simulink model "SDS_brk_cbc_v1"  (R2018b)
settings: Solver=ode1  StartTime=0.0  StopTime=Inf  FixedStep=0.001  RelTol=1e-3
PostLoadFcn:
  | , if any(exist('dsrtsu_mdlpostloadfcn', 'file') == [2, 3, 6]), try dsrtsu_mdlpostloadfcn('Execute', bdroot); catch fprintf('Error in PostLoadFcn (dsrtsu_mdlpostloadfcn) for model "%s":\n %s\n', bdroot, lasterr); end, end,
libraries: rtican x11, simulink x5
(part 3 of 4)

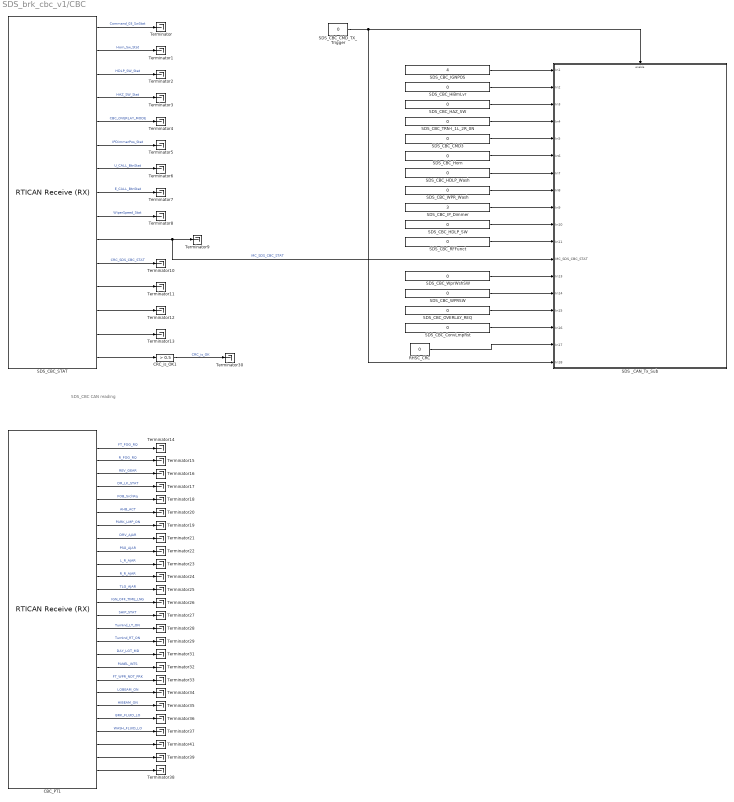
== system SDS_brk_cbc_v1/CBC ==
  note: SDS_CBC CAN reading
  CBC_PT1 : rtican/RTICAN Receive (RX)   Reserved1=[]  Reserved2=[]  Reserved3=[]  Reserved4=[]  SfcnMessage=[]  Msg_Struct=[]  BoardTypeNo=[]  BoardNo=[]  ChannelNo=[]  Parameters=[]  DialogFcn=[]  UnitName=[]  Revision=[]  UnitValues=[]  DSProperties=struct('RTI',struct('Version',uint32(5),'BlockType',struct('isSLSource',uint8(1),'isSLSink',uint8(1),'isHWSource',uint8(0),'isHWSink',uint8(0),'isSetup',uint8(0),'isInline',uint8(1),'isNonInline',uint8(0),'isInterrupt',uint8(0),'isChannelwise',uint8(0)),'IOBoardType','RTICAN','UnitType','MESSAGE','Identifier','RX','DialogType','MSVC','BlockSet','RTICAN','SlaveProcessor','CAN'))  RTIBlockInterface=struct('OutputPortsWidth',int32([1 1 1 1 1 1 1 1 1 1 1 1 1 1 1 1 1 1 1 1 1 1 1 1 1 1]),'OutputPortsActive',ones(1,26),'OutputPortsName',{{'FT_FOG_RQ','R_FOG_RQ','REV_GEAR','DR_LK_STAT','FOB_SrchRq','AHB_ACT','PARK_LMP_ON','DRV_AJAR','PSG_AJAR','L_R_AJAR','R_R_AJAR','TLG_AJAR','IGN_OFF_TIME_LNG','SHIP_STAT','TurnInd_LT_ON','TurnInd_RT_ON','DAY_LGT_MD','PANEL_INTS','FT_WPR_NOT_PRK','LOBEAM_ON','HIBEAM_ON','BRK_FLUID_LO','WASH_FLUID_LO',['RX status'],['RX time'],['RX delta time']}},'OutputPortsDataType',{{'SS_DOUBLE','SS_DOUBLE','SS_DOUBLE','SS_DOUBLE','SS_DOUBLE','SS_DOUBLE','SS_DOUBLE','SS_DOUBLE','SS_DOUBLE','SS_DOUBLE','SS_DOUBLE','SS_DOUBLE','SS_DOUBLE','SS_DOUBLE','SS_DOUBLE','SS_DOUBLE','SS_DOUBLE','SS_DOUBLE','SS_DOUBLE','SS_DOUBLE','SS_DOUBLE','SS_DOUBLE','SS_DOUBLE','SS_DOUBLE','SS_DOUBLE','SS_DOUBLE'}},'OutputPortsLabel',{{'FT_FOG_RQ','R_FOG_RQ','REV_GEAR','DR_LK_STAT','FOB_SrchRq','AHB_ACT','PARK_LMP_ON','DRV_AJAR','PSG_AJAR','L_R_AJAR','R_R_AJAR','TLG_AJAR','IGN_OFF_TIME_LNG','SHIP_STAT','TurnInd_LT_ON','TurnInd_RT_ON','DAY_LGT_MD','PANEL_INTS','FT_WPR_NOT_PRK','LOBEAM_ON','HIBEAM_ON','BRK_FLUID_LO','WASH_FLUID_LO','','',''}},'OutputPortsLabelMode','ON','InputPortsWidth',int32(0),'InputPortsActive',0,'DialogFcn','rtican_message_interface_gui','BlockDisplay',{{'','center'}},'IconTransparency','on','ParameterTunableNames',{{}},'InitLevel',3,'BlockName',struct('Token',{{'CBC_PT1'}}),'SampleTime',{{0}},'TriggerPort',{{'none'}},'EnablePort',{{'none'}})  RTIBlockParameters=struct('BoardTypeNo',{{1,'OFF',[]}},'BoardNo',{{1,'ON',[1 16]}},'ChannelNo',{{1,'ON',[1 2]}},'Parameters',{{struct('DataFileSupport',struct('DataFileSelectedMaster',1,'DataFileSelectedLocal',1,'DataFileName',['c:\intrepidcs\pacifica dbc\e4a_r4_ccan_cr11690_mod.dbc|'],'DataFileDate',{{{['26-Feb-2019 09:25:05']}}},'SelectedFile',['..\..\..\..\..\intrepidcs\pacifica dbc\e4a_r4_ccan_cr11690_mod.dbc']),'Options',struct('StatusSelected',1,'TimeSelected',1,'DeltaTimeSelected',1,'BytePortSelected',0,'MessageLengthSelected',0,'TriggerPort',struct('Selected',0,'TriggerType',0),'UserCoding',struct('Selected',0,'InterfaceFile','UserDecodingFile','FcnName','Message_CRC_Decoder','InportSelected',0,'InportWidth',1,'OutportSelected',1,'OutportWidth',1),'EnablePortSelected',0,'SignalOnPortnameSelected',1,'UseRXService',0),'Message',struct('MsgOnBlocknameSelected',1,'MsgName','CBC_PT1','MsgIdFormat',0,'MsgId',820,'MsgLength',8,'NumSignals',23,'SampleTime',0,'Signal',struct('SgnName',{'FT_FOG_RQ','R_FOG_RQ','REV_GEAR','DR_LK_STAT','FOB_SrchRq','AHB_ACT','PARK_LMP_ON','DRV_AJAR','PSG_AJAR','L_R_AJAR','R_R_AJAR','TLG_AJAR','IGN_OFF_TIME_LNG','SHIP_STAT','TurnInd_LT_ON','TurnInd_RT_ON','DAY_LGT_MD','PANEL_INTS','FT_WPR_NOT_PRK','LOBEAM_ON','HIBEAM_ON','BRK_FLUID_LO','WASH_FLUID_LO'},'SgnStartBit',{2,3,4,5,8,14,16,17,18,19,20,22,24,28,30,31,40,48,56,57,58,62,63},'SgnLength',{1,1,1,2,2,1,1,1,1,1,1,1,12,2,1,1,1,8,1,1,1,1,1},'SgnType',{0,0,0,0,0,0,0,0,0,0,0,0,0,0,0,0,0,0,0,0,0,0,0},'ModeValue',{-1,-1,-1,-1,-1,-1,-1,-1,-1,-1,-1,-1,-1,-1,-1,-1,-1,-1,-1,-1,-1,-1,-1},'DataType',{0,0,0,0,0,0,0,0,0,0,0,0,0,0,0,0,0,0,0,0,0,0,0},'ByteLayout',{0,0,0,0,0,0,0,0,0,0,0,0,2,0,0,0,0,0,0,0,0,0,0},'Factor',{1,1,1,1,1,1,1,1,1,1,1,1,1,1,1,1,1,2^-1,1,1,1,1,1},'Offset',{0,0,0,0,0,0,0,0,0,0,0,0,0,0,0,0,0,0,0,0,0,0,0},'SgnComment',{{['Front fog request; off=[0], on=[1]']},{['Rear fog request; [0] = off, [1] = on']},{['Reverse Gear (manual trans)']},{['Door lock status']},{['FOB search request']},{['Automatic high beam active']},{['Parklamps are on; off=[0], on=[1]']},{['Driver door ajar (1 = Door Ajar)']},{['Passenger door ajar']},{['Left rear door ajar']},{['Right rear door ajar']},{['Trunk/Liftgate ajar']},{['Time since last ignition on (long)']},{['Shipping status']},{['Turn indication left is on']},{['Turn indication right is on']},{['Day light brightness mode; Night=[0], Day=[1]']},{['Panel-/display intensity']},{['Front wiper outside park position']},{['Low beam is on; off=[0], on=[1]']},{['High beam is on; off=[0], on=[1]']},{['Low brake fluid warning; low = [1]']},{['Low washer fluid warning (1=Fluid is low)']}},'SgnUnit',{'','','','','','','','','','','','','min','','','','','%','','','','',''},'Min',{0,0,0,0,0,0,0,0,0,0,0,0,0,0,0,0,0,0,0,0,0,0,0},'Max',{0,0,0,0,0,0,0,0,0,0,0,0,4080,0,0,0,0,100,0,0,0,0,0},'SLDataType',{'SS_DOUBLE','SS_DOUBLE','SS_DOUBLE','SS_DOUBLE','SS_DOUBLE','SS_DOUBLE','SS_DOUBLE','SS_DOUBLE','SS_DOUBLE','SS_DOUBLE','SS_DOUBLE','SS_DOUBLE','SS_DOUBLE','SS_DOUBLE','SS_DOUBLE','SS_DOUBLE','SS_DOUBLE','SS_DOUBLE','SS_DOUBLE','SS_DOUBLE','SS_DOUBLE','SS_DOUBLE','SS_DOUBLE'}),'MsgIdNumFormat',0,'MsgComment',{{''}}),'Version',1.2,'general',struct('isFromLib',0)),'OFF',[]}},'GroupId',{{struct('Group',{{'RTICAN'}},'No',1,'Behavior',{{'NAMECHANGE'}},'BlockType',{{'SINK'}},'NameChangeFlag',0),'OFF',[]}},'SFcnRTICANMessage',{{struct('MsgType','RX','SFcnPortType','Scalar','MsgName','CBC_PT1','MsgIdFormat','STD','MsgId',820,'MsgLength',8,'NumSignals',23,'SampleTime',0,'Signal',struct('SgnName',{'FT_FOG_RQ','R_FOG_RQ','REV_GEAR','DR_LK_STAT','FOB_SrchRq','AHB_ACT','PARK_LMP_ON','DRV_AJAR','PSG_AJAR','L_R_AJAR','R_R_AJAR','TLG_AJAR','IGN_OFF_TIME_LNG','SHIP_STAT','TurnInd_LT_ON','TurnInd_RT_ON','DAY_LGT_MD','PANEL_INTS','FT_WPR_NOT_PRK','LOBEAM_ON','HIBEAM_ON','BRK_FLUID_LO','WASH_FLUID_LO'},'SgnStartBit',{2,3,4,5,8,14,16,17,18,19,20,22,24,28,30,31,40,48,56,57,58,62,63},'SgnLength',{1,1,1,2,2,1,1,1,1,1,1,1,12,2,1,1,1,8,1,1,1,1,1},'SgnType',{'standard','standard','standard','standard','standard','standard','standard','standard','standard','standard','standard','standard','standard','standard','standard','standard','standard','standard','standard','standard','standard','standard','standard'},'ModeValue',{-1,-1,-1,-1,-1,-1,-1,-1,-1,-1,-1,-1,-1,-1,-1,-1,-1,-1,-1,-1,-1,-1,-1},'DataType',{['unsigned int'],['unsigned int'],['unsigned int'],['unsigned int'],['unsigned int'],['unsigned int'],['unsigned int'],['unsigned int'],['unsigned int'],['unsigned int'],['unsigned int'],['unsigned int'],['unsigned int'],['unsigned int'],['unsigned int'],['unsigned int'],['unsigned int'],['unsigned int'],['unsigned int'],['unsigned int'],['unsigned int'],['unsigned int'],['unsigned int']},'ByteLayout',{['little endian'],['little endian'],['little endian'],['little endian'],['little endian'],['little endian'],['little endian'],['little endian'],['little endian'],['little endian'],['little endian'],['little endian'],['motorola back.'],['little endian'],['little endian'],['little endian'],['little endian'],['little endian'],['little endian'],['little endian'],['little endian'],['little endian'],['little endian']},'Factor',{1,1,1,1,1,1,1,1,1,1,1,1,1,1,1,1,1,2^-1,1,1,1,1,1},'Offset',{0,0,0,0,0,0,0,0,0,0,0,0,0,0,0,0,0,0,0,0,0,0,0},'SLDataType',{'SS_DOUBLE','SS_DOUBLE','SS_DOUBLE','SS_DOUBLE','SS_DOUBLE','SS_DOUBLE','SS_DOUBLE','SS_DOUBLE','SS_DOUBLE','SS_DOUBLE','SS_DOUBLE','SS_DOUBLE','SS_DOUBLE','SS_DOUBLE','SS_DOUBLE','SS_DOUBLE','SS_DOUBLE','SS_DOUBLE','SS_DOUBLE','SS_DOUBLE','SS_DOUBLE','SS_DOUBLE','SS_DOUBLE'}),'StatusSelected','yes','TimeSelected','yes','DeltaTimeSelected','yes','BytePortSelected','no','MessageLengthSelected','no','TriggerPort',struct('Selected','no','TriggerType',0),'UserCoding',struct('Selected','no','InterfaceFile','UserDecodingFile','FcnName','Message_CRC_Decoder','InportSelected','no','InportWidth',1,'OutportSelected','yes','OutportWidth',1),'EnablePortSelected','no','UseRXService','no','BoardType','DS1','BoardNo',1,'ControllerNo',1),'OFF',[]}},'TLCFileName',{{'rtican_rx_message','OFF',[]}})  RTISFcnParameters=struct('SFcnRTICANMessage','struct','TLCFileName','char')  RTIBlockParaDefault=struct('BoardTypeNo',4302,'BoardNo',1,'ChannelNo',1,'Parameters',struct('DataFileSupport',struct('DataFileSelectedMaster',0,'DataFileSelectedLocal',0,'DataFileName','','DataFileDate','','SelectedFile',['<no file selected>']),'Options',struct('StatusSelected',1,'TimeSelected',1,'DeltaTimeSelected',1,'BytePortSelected',0,'MessageLengthSelected',0,'TriggerPort',struct('Selected',0,'TriggerType','rising'),'UserCoding',struct('Selected',0,'InterfaceFile','UserDecodingFile','FcnName','UserDecodeFcn','InportSelected',0,'InportWidth',1,'OutportSelected',0,'OutportWidth',1),'EnablePortSelected',0,'SignalOnPortnameSelected',1,'UseRXService',0),'Message',struct('MsgOnBlocknameSelected',0,'MsgName',['RX Message'],'MsgIdFormat',0,'MsgId',100,'MsgLength',8,'NumSignals',1,'SampleTime',-1,'Signal',struct('SgnName',['RX signal'],'SgnStartBit',0,'SgnLength',8,'SgnType',0,'ModeValue',-1,'DataType',0,'SLDataType','SS_DOUBLE','ByteLayout',0,'Factor',1,'Offset',0,'Min',0,'Max',255,'SgnComment',{{}},'SgnUnit',''),'MsgIdNumFormat',0,'MsgComment',{{''}}),'Version',1.2,'general',struct('isFromLib',1)),'GroupId',struct('Group',{{'RTICAN'}},'No',1,'Behavior',{{'NAMECHANGE'}},'BlockType',{{'SINK'}},'NameChangeFlag',0),'SFcnRTICANMessage',struct('MsgType','RX','MsgName',['RX Message'],'MsgIdFormat','STD','MsgId',100,'MsgLength',8,'NumSignals',1,'SampleTime',-1,'Signal',struct('SgnName',['RX signal'],'SgnStartBit',0,'SgnLength',8,'SgnType','standard','ModeValue',-1,'DataType',['unsigned int'],'ByteLayout',['little endian'],'SLDataType','SS_DOUBLE','Factor',1,'Offset',0),'StatusSelected','yes','TimeSelected','yes','DeltaTimeSelected','yes','BytePortSelected','no','MessageLengthSelected','no','EnablePortSelected','no','UserCoding',struct('Selected','no','InterfaceFile','UserDecodingFile','FcnName','UserDecodeFcn','InportSelected','no','InportWidth',1,'OutportSelected','no','OutportWidth',1),'TriggerPort',struct('Selected','no','TriggerType','rising'),'UseRXService','no','BoardType','DS4302','BoardNo',1,'ControllerNo',1,'SFcnPortType','Scalar'),'TLCFileName','rtican_rx_message')
      settings: AttributesFormatString=Group Id: RTICAN1\n  SourceProductName=dSPACE RTI CAN Blockset
  CRC_is_OK1 : simulink/Logic and Bit Operations/Compare To Constant  relop=>  const=0.5  OutDataTypeStr=boolean
  RHSC_CRC : Constant  Value=0  OutDataTypeStr=Inherit: Inherit via back propagation
  "SDS _CAN_Tx_Sub " : Subsystem
  SDS_CBC_CMD3 : Constant  Value=0
  SDS_CBC_CMD_TX_Trigger : Constant  Value=0  OutDataTypeStr=Inherit: Inherit via back propagation
  SDS_CBC_ConvLmpRst : Constant  Value=0
  SDS_CBC_HAZ_SW : Constant  Value=0
  SDS_CBC_HDLP_SW : Constant  Value=0
  SDS_CBC_HDLP_Wash : Constant  Value=0
  SDS_CBC_HiBmLvr : Constant  Value=0
  SDS_CBC_Horn : Constant  Value=0
  SDS_CBC_IGNPOS : Constant  Value=4  OutMin=0  OutMax=6
  SDS_CBC_IP_Dimmer : Constant  Value=3
  SDS_CBC_OVERLAY_REQ : Constant  Value=0
  SDS_CBC_RFFunct : Constant  Value=0
  SDS_CBC_STAT : rtican/RTICAN Receive (RX)   Reserved1=[]  Reserved2=[]  Reserved3=[]  Reserved4=[]  SfcnMessage=[]  Msg_Struct=[]  BoardTypeNo=[]  BoardNo=[]  ChannelNo=[]  Parameters=[]  DialogFcn=[]  UnitName=[]  Revision=[]  UnitValues=[]  DSProperties=struct('RTI',struct('Version',uint32(5),'BlockType',struct('isSLSource',uint8(1),'isSLSink',uint8(1),'isHWSource',uint8(0),'isHWSink',uint8(0),'isSetup',uint8(0),'isInline',uint8(1),'isNonInline',uint8(0),'isInterrupt',uint8(0),'isChannelwise',uint8(0)),'IOBoardType','RTICAN','UnitType','MESSAGE','Identifier','RX','DialogType','MSVC','BlockSet','RTICAN','SlaveProcessor','CAN'))  RTIBlockInterface=struct('OutputPortsWidth',int32([1 1 1 1 1 1 1 1 1 1 1 1 1 1 1]),'OutputPortsActive',ones(1,15),'OutputPortsName',{{'Command_03_SwStat','Horn_Sw_Stat','HDLP_SW_Stat','HAZ_SW_Stat','CBC_OVERLAY_MODE','IPDimmerPos_Stat','U_CALL_BtnStat','E_CALL_BtnStat','WiperSpeed_Stat','MC_SDS_CBC_STAT','CRC_SDS_CBC_STAT',['RX status'],['RX time'],['RX delta time'],['User outport']}},'OutputPortsDataType',{{'SS_DOUBLE','SS_DOUBLE','SS_DOUBLE','SS_DOUBLE','SS_DOUBLE','SS_DOUBLE','SS_DOUBLE','SS_DOUBLE','SS_DOUBLE','SS_DOUBLE','SS_DOUBLE','SS_DOUBLE','SS_DOUBLE','SS_DOUBLE','SS_DOUBLE'}},'OutputPortsLabel',{{'Command_03_SwStat','Horn_Sw_Stat','HDLP_SW_Stat','HAZ_SW_Stat','CBC_OVERLAY_MODE','IPDimmerPos_Stat','U_CALL_BtnStat','E_CALL_BtnStat','WiperSpeed_Stat','MC_SDS_CBC_STAT','CRC_SDS_CBC_STAT','','','',''}},'OutputPortsLabelMode','ON','InputPortsWidth',int32(0),'InputPortsActive',0,'DialogFcn','rtican_message_interface_gui','BlockDisplay',{{'','center'}},'IconTransparency','on','ParameterTunableNames',{{}},'InitLevel',3,'BlockName',struct('Token',{{'SDS_CBC_STAT'}}),'SampleTime',{{0}},'TriggerPort',{{'none'}},'EnablePort',{{'none'}})  RTIBlockParameters=struct('BoardTypeNo',{{1,'OFF',[]}},'BoardNo',{{1,'ON',[1 16]}},'ChannelNo',{{1,'ON',[1 2]}},'Parameters',{{struct('DataFileSupport',struct('DataFileSelectedMaster',1,'DataFileSelectedLocal',1,'DataFileName',['c:\intrepidcs\pacifica dbc\e4a_r4_ccan_cr11690_mod.dbc|'],'DataFileDate',{{{['26-Feb-2019 09:25:05']}}},'SelectedFile',['..\..\..\..\..\intrepidcs\pacifica dbc\e4a_r4_ccan_cr11690_mod.dbc']),'Options',struct('StatusSelected',1,'TimeSelected',1,'DeltaTimeSelected',1,'BytePortSelected',0,'MessageLengthSelected',0,'TriggerPort',struct('Selected',0,'TriggerType',0),'UserCoding',struct('Selected',1,'InterfaceFile','UserDecodingFile','FcnName','Message_CRC_Decoder','InportSelected',0,'InportWidth',1,'OutportSelected',1,'OutportWidth',1),'EnablePortSelected',0,'SignalOnPortnameSelected',1,'UseRXService',0),'Message',struct('MsgOnBlocknameSelected',1,'MsgName','SDS_CBC_STAT','MsgIdFormat',0,'MsgId',858,'MsgLength',5,'NumSignals',11,'SampleTime',0,'Signal',struct('SgnName',{'Command_03_SwStat','Horn_Sw_Stat','HDLP_SW_Stat','HAZ_SW_Stat','CBC_OVERLAY_MODE','IPDimmerPos_Stat','U_CALL_BtnStat','E_CALL_BtnStat','WiperSpeed_Stat','MC_SDS_CBC_STAT','CRC_SDS_CBC_STAT'},'SgnStartBit',{0,2,4,7,13,16,20,22,24,28,32},'SgnLength',{2,1,3,1,3,4,2,2,2,4,8},'SgnType',{0,0,0,0,0,0,0,0,0,0,0},'ModeValue',{-1,-1,-1,-1,-1,-1,-1,-1,-1,-1,-1},'DataType',{0,0,0,0,0,0,0,0,0,0,0},'ByteLayout',{0,0,0,0,0,0,0,0,0,0,0},'Factor',{1,1,1,1,1,1,1,1,1,1,1},'Offset',{0,0,0,0,0,0,0,0,0,0,0},'SgnComment',{{['Steering wheel switch 3 - Actual Switch Status (mode button)']},{['Physical Horn Pad Status']},{['Headlamp switch actual status']},{['Hazard Switch Actual Status; Not Pressed = [0], Pressed = [1];']},{['CBC Overlay Mode']},{['IP Dimmer Position Status to RHSC2']},{['Ucall button status to RHSC2']},{['Ecall button status to RHSC2']},{['Speed of wiper from RLS']},{['Message counter']},{['CRC-checksum byte 1 to 4 according to SAE J1850']}},'SgnUnit',{'','','','','','','','','','',''},'Min',{0,0,0,0,0,0,0,0,0,0,0},'Max',{0,0,0,0,0,0,0,0,0,15,0},'SLDataType',{'SS_DOUBLE','SS_DOUBLE','SS_DOUBLE','SS_DOUBLE','SS_DOUBLE','SS_DOUBLE','SS_DOUBLE','SS_DOUBLE','SS_DOUBLE','SS_DOUBLE','SS_DOUBLE'}),'MsgIdNumFormat',0,'MsgComment',{{''}}),'Version',1.2,'general',struct('isFromLib',0)),'OFF',[]}},'GroupId',{{struct('Group',{{'RTICAN'}},'No',1,'Behavior',{{'NAMECHANGE'}},'BlockType',{{'SINK'}},'NameChangeFlag',0),'OFF',[]}},'SFcnRTICANMessage',{{struct('MsgType','RX','SFcnPortType','Scalar','MsgName','SDS_CBC_STAT','MsgIdFormat','STD','MsgId',858,'MsgLength',5,'NumSignals',11,'SampleTime',0,'Signal',struct('SgnName',{'Command_03_SwStat','Horn_Sw_Stat','HDLP_SW_Stat','HAZ_SW_Stat','CBC_OVERLAY_MODE','IPDimmerPos_Stat','U_CALL_BtnStat','E_CALL_BtnStat','WiperSpeed_Stat','MC_SDS_CBC_STAT','CRC_SDS_CBC_STAT'},'SgnStartBit',{0,2,4,7,13,16,20,22,24,28,32},'SgnLength',{2,1,3,1,3,4,2,2,2,4,8},'SgnType',{'standard','standard','standard','standard','standard','standard','standard','standard','standard','standard','standard'},'ModeValue',{-1,-1,-1,-1,-1,-1,-1,-1,-1,-1,-1},'DataType',{['unsigned int'],['unsigned int'],['unsigned int'],['unsigned int'],['unsigned int'],['unsigned int'],['unsigned int'],['unsigned int'],['unsigned int'],['unsigned int'],['unsigned int']},'ByteLayout',{['little endian'],['little endian'],['little endian'],['little endian'],['little endian'],['little endian'],['little endian'],['little endian'],['little endian'],['little endian'],['little endian']},'Factor',{1,1,1,1,1,1,1,1,1,1,1},'Offset',{0,0,0,0,0,0,0,0,0,0,0},'SLDataType',{'SS_DOUBLE','SS_DOUBLE','SS_DOUBLE','SS_DOUBLE','SS_DOUBLE','SS_DOUBLE','SS_DOUBLE','SS_DOUBLE','SS_DOUBLE','SS_DOUBLE','SS_DOUBLE'}),'StatusSelected','yes','TimeSelected','yes','DeltaTimeSelected','yes','BytePortSelected','no','MessageLengthSelected','no','TriggerPort',struct('Selected','no','TriggerType',0),'UserCoding',struct('Selected','yes','InterfaceFile','UserDecodingFile','FcnName','Message_CRC_Decoder','InportSelected','no','InportWidth',1,'OutportSelected','yes','OutportWidth',1),'EnablePortSelected','no','UseRXService','no','BoardType','DS1','BoardNo',1,'ControllerNo',1),'OFF',[]}},'TLCFileName',{{'rtican_rx_message','OFF',[]}})  RTISFcnParameters=struct('SFcnRTICANMessage','struct','TLCFileName','char')  RTIBlockParaDefault=struct('BoardTypeNo',4302,'BoardNo',1,'ChannelNo',1,'Parameters',struct('DataFileSupport',struct('DataFileSelectedMaster',0,'DataFileSelectedLocal',0,'DataFileName','','DataFileDate','','SelectedFile',['<no file selected>']),'Options',struct('StatusSelected',1,'TimeSelected',1,'DeltaTimeSelected',1,'BytePortSelected',0,'MessageLengthSelected',0,'TriggerPort',struct('Selected',0,'TriggerType','rising'),'UserCoding',struct('Selected',0,'InterfaceFile','UserDecodingFile','FcnName','UserDecodeFcn','InportSelected',0,'InportWidth',1,'OutportSelected',0,'OutportWidth',1),'EnablePortSelected',0,'SignalOnPortnameSelected',1,'UseRXService',0),'Message',struct('MsgOnBlocknameSelected',0,'MsgName',['RX Message'],'MsgIdFormat',0,'MsgId',100,'MsgLength',8,'NumSignals',1,'SampleTime',-1,'Signal',struct('SgnName',['RX signal'],'SgnStartBit',0,'SgnLength',8,'SgnType',0,'ModeValue',-1,'DataType',0,'SLDataType','SS_DOUBLE','ByteLayout',0,'Factor',1,'Offset',0,'Min',0,'Max',255,'SgnComment',{{}},'SgnUnit',''),'MsgIdNumFormat',0,'MsgComment',{{''}}),'Version',1.2,'general',struct('isFromLib',1)),'GroupId',struct('Group',{{'RTICAN'}},'No',1,'Behavior',{{'NAMECHANGE'}},'BlockType',{{'SINK'}},'NameChangeFlag',0),'SFcnRTICANMessage',struct('MsgType','RX','MsgName',['RX Message'],'MsgIdFormat','STD','MsgId',100,'MsgLength',8,'NumSignals',1,'SampleTime',-1,'Signal',struct('SgnName',['RX signal'],'SgnStartBit',0,'SgnLength',8,'SgnType','standard','ModeValue',-1,'DataType',['unsigned int'],'ByteLayout',['little endian'],'SLDataType','SS_DOUBLE','Factor',1,'Offset',0),'StatusSelected','yes','TimeSelected','yes','DeltaTimeSelected','yes','BytePortSelected','no','MessageLengthSelected','no','EnablePortSelected','no','UserCoding',struct('Selected','no','InterfaceFile','UserDecodingFile','FcnName','UserDecodeFcn','InportSelected','no','InportWidth',1,'OutportSelected','no','OutportWidth',1),'TriggerPort',struct('Selected','no','TriggerType','rising'),'UseRXService','no','BoardType','DS4302','BoardNo',1,'ControllerNo',1,'SFcnPortType','Scalar'),'TLCFileName','rtican_rx_message')
      settings: AttributesFormatString=Group Id: RTICAN1\n  SourceProductName=dSPACE RTI CAN Blockset
  SDS_CBC_TRN-I_1L_2R_0N : Constant  Value=0
  SDS_CBC_WPRSW : Constant  Value=0
  SDS_CBC_WPR_Wash : Constant  Value=0
  SDS_CBC_WprWshSW : Constant  Value=0
  Terminator{,1..39,41} (41 alike) : Terminator
  wires:
  SDS_CBC_STAT/13 -> Terminator12/1
  CBC_PT1/6 -> Terminator20/1  "AHB_ACT"
  SDS_CBC_STAT/7 -> Terminator6/1  "U_CALL_BtnStat"
  SDS_CBC_STAT/11 -> Terminator10/1  "CRC_SDS_CBC_STAT"
  SDS_CBC_STAT/2 -> Terminator1/1  "Horn_Sw_Stat"
  SDS_CBC_CMD_TX_Trigger/1 -> "SDS _CAN_Tx_Sub "/18(In18), "SDS _CAN_Tx_Sub "/Enable
  CBC_PT1/11 -> Terminator24/1  "R_R_AJAR"
  SDS_CBC_TRN-I_1L_2R_0N/1 -> "SDS _CAN_Tx_Sub "/4(In4)
  SDS_CBC_STAT/8 -> Terminator7/1  "E_CALL_BtnStat"
  CBC_PT1/25 -> Terminator39/1
  SDS_CBC_WPRSW/1 -> "SDS _CAN_Tx_Sub "/14(In14)
  SDS_CBC_ConvLmpRst/1 -> "SDS _CAN_Tx_Sub "/16(In16)
  SDS_CBC_STAT/9 -> Terminator8/1  "WiperSpeed_Stat"
  SDS_CBC_STAT/12 -> Terminator11/1
  SDS_CBC_OVERLAY_REQ/1 -> "SDS _CAN_Tx_Sub "/15(In15)
  CBC_PT1/23 -> Terminator37/1  "WASH_FLUID_LO"
  SDS_CBC_STAT/5 -> Terminator4/1  "CBC_OVERLAY_MODE"
  CBC_PT1/4 -> Terminator17/1  "DR_LK_STAT"
  RHSC_CRC/1 -> "SDS _CAN_Tx_Sub "/17(In17)
  CBC_PT1/18 -> Terminator32/1  "PANEL_INTS"
  SDS_CBC_STAT/3 -> Terminator2/1  "HDLP_SW_Stat"
  CBC_PT1/3 -> Terminator16/1  "REV_GEAR"
  SDS_CBC_IGNPOS/1 -> "SDS _CAN_Tx_Sub "/1(In1)
  CBC_PT1/14 -> Terminator27/1  "SHIP_STAT"
  CBC_PT1/15 -> Terminator28/1  "TurnInd_LT_ON"
  SDS_CBC_WPR_Wash/1 -> "SDS _CAN_Tx_Sub "/8(In8)
  SDS_CBC_STAT/10 -> "SDS _CAN_Tx_Sub "/12(MC_SDS_CBC_STAT), Terminator9/1  "MC_SDS_CBC_STAT"
  SDS_CBC_WprWshSW/1 -> "SDS _CAN_Tx_Sub "/13(In13)
  CBC_PT1/26 -> Terminator38/1
  CBC_PT1/24 -> Terminator41/1
  SDS_CBC_STAT/14 -> Terminator13/1
  CBC_PT1/9 -> Terminator22/1  "PSG_AJAR"
  CBC_PT1/5 -> Terminator18/1  "FOB_SrchRq"
  SDS_CBC_STAT/4 -> Terminator3/1  "HAZ_SW_Stat"
  SDS_CBC_HDLP_SW/1 -> "SDS _CAN_Tx_Sub "/10(In10)
  SDS_CBC_STAT/6 -> Terminator5/1  "IPDimmerPos_Stat"
  CBC_PT1/21 -> Terminator35/1  "HIBEAM_ON"
  CBC_PT1/22 -> Terminator36/1  "BRK_FLUID_LO"
  SDS_CBC_STAT/1 -> Terminator/1  "Command_03_SwStat"
  SDS_CBC_Horn/1 -> "SDS _CAN_Tx_Sub "/6(In6)
  CBC_PT1/1 -> Terminator14/1  "FT_FOG_RQ"
  CBC_PT1/8 -> Terminator21/1  "DRV_AJAR"
  SDS_CBC_HiBmLvr/1 -> "SDS _CAN_Tx_Sub "/2(In2)
  SDS_CBC_RFFunct/1 -> "SDS _CAN_Tx_Sub "/11(In11)
  SDS_CBC_HDLP_Wash/1 -> "SDS _CAN_Tx_Sub "/7(In7)
  CBC_PT1/20 -> Terminator34/1  "LOBEAM_ON"
  CBC_PT1/19 -> Terminator33/1  "FT_WPR_NOT_PRK"
  CBC_PT1/2 -> Terminator15/1  "R_FOG_RQ"
  SDS_CBC_CMD3/1 -> "SDS _CAN_Tx_Sub "/5(In5)
  CBC_PT1/13 -> Terminator26/1  "IGN_OFF_TIME_LNG"
  CBC_PT1/10 -> Terminator23/1  "L_R_AJAR"
  CBC_PT1/7 -> Terminator19/1  "PARK_LMP_ON"
  CBC_PT1/17 -> Terminator31/1  "DAY_LGT_MD"
  SDS_CBC_HAZ_SW/1 -> "SDS _CAN_Tx_Sub "/3(In3)
  CBC_PT1/16 -> Terminator29/1  "TurnInd_RT_ON"
  SDS_CBC_STAT/15 -> CRC_is_OK1/1
  CRC_is_OK1/1 -> Terminator30/1  "CRC_is_OK"
  SDS_CBC_IP_Dimmer/1 -> "SDS _CAN_Tx_Sub "/9(In9)
  CBC_PT1/12 -> Terminator25/1  "TLG_AJAR"

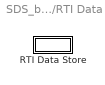
== system SDS_brk_cbc_v1/RTI Data ==
  RTI Data Store : Subsystem  Tag="struct('private',struct('version',struct('dsVer',uint32(2),'dsVerCreation',uint32(2),'RTI',struct('ver','7.10','type','RTI1401')),'access',struct('type','Model','isPerm',1,'created',['24-Apr-2019 12:45:49'],'modified',['02-Oct-2019 13:55:59'],'location','')),'public',struct('main',struct('data',[]),'sub',struct('name',{{'SDS_brk_cbc_v1'}},'data',{{struct('TH',struct('thTaskInfo',struct('taskType',{'TIMER','HWINT','TMRINT','SWINT','GLINT'},'tasksNumOf',{1,0,0,0,0},'srcIds',{{'TIMERA'},{},{},{},{}},'taskNames',{{['Timer Task 1']},{},{},{},{}})),'th_tc',struct('dataType','TASK','taskGroupId','','taskGroupList',{{}},'taskSchedulingPolicy','FCFS','taskType','TIMER','blkh',-1,'srcId','TIMERA','srcSgnName',['Timer A interrupt'],'srcCpuName','','taskName',['Timer Task 1  [0.001] s'],'taskNameDisplayExt','','smplTime',0.001,'smplTimeOffs',0,'hasFixedPriority',0,'priority',1,'hasFixedOvc',0,'ovcType',1,'ovcMax',1),'tc_th',struct('dataType','TASK','taskGroupId','','taskGroupList',{{}},'taskSchedulingPolicy','FCFS','taskType','TIMER','blkh',-1,'srcId','TIMERA','srcSgnName',['Timer A interrupt'],'srcCpuName','','taskName',['Timer Task 1  [0.001] s'],'taskNameDisplayExt','','smplTime',0.001,'smplTimeOffs',0,'hasFixedPriority',0,'priority',1,'hasFixedOvc',0,'ovcType',1,'ovcMax',1))}})))"  mask(RTI_DATA_STORE){}
      mask help:
      | RTI Data Store Block. This block is used by RTI to store internal model dependent data. Deleting this block will result in data loss.
      |
      | NEVER DELETE, COPY, OR MODIFY THIS BLOCK!
      mask Help:
      | RTI Data Store Block. This block is used by RTI to store internal model dependent data. Deleting this block will result in data loss.
      | 
      | NEVER DELETE, COPY, OR MODIFY THIS BLOCK!
      mask Display: text(0.5, 0.5, ' ', 'HorizontalAlignment', 'center');

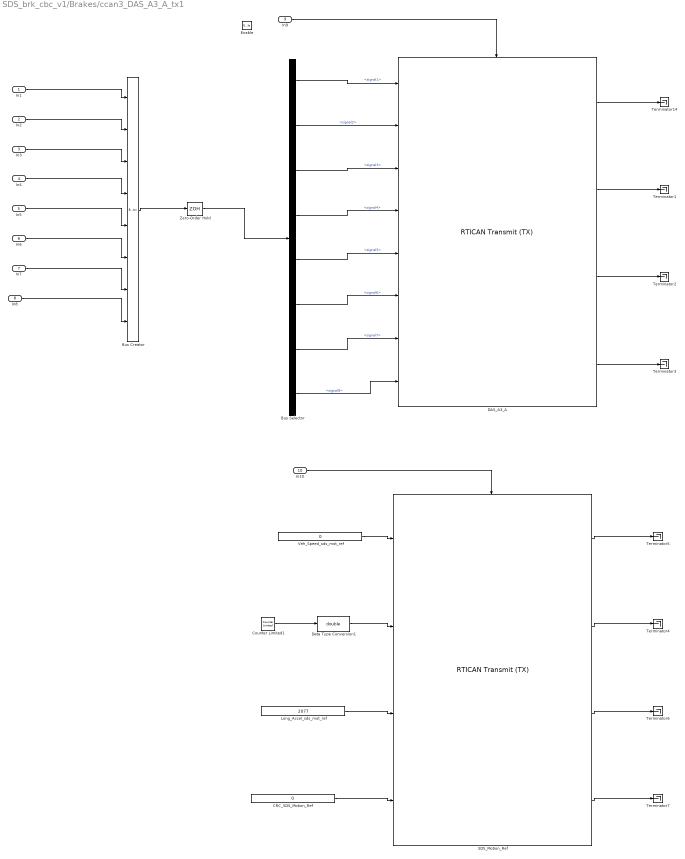
== system SDS_brk_cbc_v1/Brakes/ccan3_DAS_A3_A_tx1 ==
  In1 : Inport
  In2 : Inport  Port=2
  In3 : Inport  Port=3
  In4 : Inport  Port=4
  In5 : Inport  Port=5
  In6 : Inport  Port=6
  In7 : Inport  Port=7
  In8 : Inport  Port=8
  In9 : Inport  Port=9
  In10 : Inport  Port=10
  Enable : EnablePort
  Bus Creator : BusCreator  Inputs=8
  Bus Selector : BusSelector  OutputSignals=signal1,signal2,signal3,signal4,signal5,signal6,signal7,signal8
  CRC_SDS_Motion_Ref : Constant  Value=0  OutMin=0  OutMax=6  OutDataTypeStr=Inherit: Inherit via back propagation
  Counter Limited1 : simulink/Sources/Counter Limited  uplimit=15  tsamp=.01
  DAS_A3_A : rtican/RTICAN Transmit (TX)   Reserved1=[]  Reserved2=[]  Reserved3=[]  Reserved4=[]  SfcnMessage=[]  Msg_Struct=[]  BoardTypeNo=[]  BoardNo=[]  ChannelNo=[]  Parameters=[]  DialogFcn=[]  UnitName=[]  Revision=[]  UnitValues=[]  DSProperties=struct('RTI',struct('Version',uint32(5),'BlockType',struct('isSLSource',uint8(1),'isSLSink',uint8(1),'isHWSource',uint8(0),'isHWSink',uint8(0),'isSetup',uint8(0),'isInline',uint8(1),'isNonInline',uint8(0),'isInterrupt',uint8(0),'isChannelwise',uint8(0)),'IOBoardType','RTICAN','UnitType','MESSAGE','Identifier','TX','DialogType','MSVC','BlockSet','RTICAN','SlaveProcessor','CAN'))  RTIBlockInterface=struct('InputPortsWidth',int32([1 1 1 1 1 1 1 1]),'InputPortsActive',[1 1 1 1 1 1 1 1],'InputPortsName',{{'SDS_Engaged_State','DAS_EPB_APPLY_RQ','RHSC_OpenLoopBraking_Rq','DAS_EPB_RELSE_RQ','LFC_Request_Type','LFC_Request','MC_DAS_A3_A','CRC_DAS_A3_A'}},'InputPortsDataType',{{'SS_DOUBLE','SS_DOUBLE','SS_DOUBLE','SS_DOUBLE','SS_DOUBLE','SS_DOUBLE','SS_DOUBLE','SS_DOUBLE'}},'OutputPortsWidth',int32([1 1 1 1]),'OutputPortsActive',[1 1 1 1],'OutputPortsName',{{['TX status'],['TX time'],['TX delta time'],['TX delay time']}},'DialogFcn','rtican_message_interface_gui','BlockDisplay',{{'','center'}},'IconTransparency','on','InitLevel',3,'BlockName',struct('Token',{{'DAS_A3_A'}}),'SampleTime',{{-1}},'TriggerPort',{{'none'}},'EnablePort',{{'yes'}})  RTIBlockParameters=struct('BoardTypeNo',{{1,'OFF',[]}},'BoardNo',{{1,'ON',[1 16]}},'ChannelNo',{{2,'ON',[1 2]}},'Parameters',{{struct('DataFileSupport',struct('DataFileSelectedMaster',1,'DataFileSelectedLocal',1,'DataFileName',['c:\intrepidcs\pacifica dbc\e4a_r4_ccan3_cr11690_mod.dbc|'],'DataFileDate',{{{['26-Feb-2019 09:25:05']}}},'SelectedFile',['..\..\..\..\..\intrepidcs\pacifica dbc\e4a_r4_ccan3_cr11690_mod.dbc']),'Options',struct('StatusSelected',1,'TimeSelected',1,'DeltaTimeSelected',1,'DelayTimeSelected',1,'DelayTimeTXCommandSelected',0,'EncodeSetUnusedBitsToOne',0,'EnableMsgLoopback',0,'TriggerPort',struct('Selected',0,'TriggerType',0),'EnablePortSelected',1,'SignalOnPortnameSelected',1,'UserCoding',struct('Selected',1,'InterfaceFile','UserEncodingFile','FcnName','Message_CRC_Encoder','InportSelected',0,'InportWidth',1,'OutportSelected',0,'OutportWidth',1),'TerminationMsg',struct('Selected',0,'Byte0_7','0'),'InitialMsg',struct('Selected',0,'Byte0_7','0')),'Message',struct('MsgOnBlocknameSelected',1,'MsgName','DAS_A3_A','MsgIdFormat',0,'MsgId',499,'MsgLength',8,'NumSignals',8,'SampleTime',-1,'StartTime',struct('Selected',1,'Value',0),'AutoRepeatTime',struct('Selected',1,'Value',0.01),'Timeout',struct('Selected',0,'Value',0.1),'DelayTime',struct('Selected',0,'Value',0.1),'Signal',struct('SgnName',{'SDS_Engaged_State','DAS_EPB_APPLY_RQ','RHSC_OpenLoopBraking_Rq','DAS_EPB_RELSE_RQ','LFC_Request_Type','LFC_Request','MC_DAS_A3_A','CRC_DAS_A3_A'},'SgnStartBit',{1,3,4,5,6,17,52,56},'SgnLength',{2,1,1,1,2,15,4,8},'SgnType',{0,0,0,0,0,0,0,0},'ModeValue',{-1,-1,-1,-1,-1,-1,-1,-1},'DataType',{0,0,0,0,0,0,0,0},'ByteLayout',{0,0,0,0,0,2,0,0},'Factor',{1,1,1,1,1,2,1,1},'Offset',{0,0,0,0,0,-65534,0,0},'SgnComment',{{['SDS Engaged Status']},{['DAS request to apply EPB']},{['Longitudinal Force Control Open Loop Braking Request']},{['DAS request to release EPB']},{['Longitudinal Force Control Request Type']},{''},{''},{''}},'SgnUnit',{'','','','','','','',''},'Min',{0,0,0,0,0,-65534,0,0},'Max',{0,0,0,0,0,0,15,255},'SLDataType',{'SS_DOUBLE','SS_DOUBLE','SS_DOUBLE','SS_DOUBLE','SS_DOUBLE','SS_DOUBLE','SS_DOUBLE','SS_DOUBLE'}),'MsgIdNumFormat',0,'MsgComment',{{''}}),'Version',1.2,'general',struct('isFromLib',0)),'OFF',[]}},'GroupId',{{struct('Group',{{'RTICAN'}},'No',2,'Behavior',{{'NAMECHANGE'}},'BlockType',{{'SINK'}},'NameChangeFlag',0),'OFF',[]}},'SFcnRTICANMessage',{{struct('MsgType','TX','SFcnPortType','Scalar','MsgName','DAS_A3_A','MsgIdFormat','STD','MsgId',499,'MsgLength',8,'NumSignals',8,'SampleTime',-1,'StartTime',struct('Selected','yes','Value',0),'AutoRepeatTime',struct('Selected','yes','Value',0.01),'Timeout',struct('Selected','no','Value',0.1),'Signal',struct('SgnName',{'SDS_Engaged_State','DAS_EPB_APPLY_RQ','RHSC_OpenLoopBraking_Rq','DAS_EPB_RELSE_RQ','LFC_Request_Type','LFC_Request','MC_DAS_A3_A','CRC_DAS_A3_A'},'SgnStartBit',{1,3,4,5,6,17,52,56},'SgnLength',{2,1,1,1,2,15,4,8},'SgnType',{'standard','standard','standard','standard','standard','standard','standard','standard'},'ModeValue',{-1,-1,-1,-1,-1,-1,-1,-1},'DataType',{['unsigned int'],['unsigned int'],['unsigned int'],['unsigned int'],['unsigned int'],['unsigned int'],['unsigned int'],['unsigned int']},'ByteLayout',{['little endian'],['little endian'],['little endian'],['little endian'],['little endian'],['motorola back.'],['little endian'],['little endian']},'Factor',{1,1,1,1,1,2,1,1},'Offset',{0,0,0,0,0,-65534,0,0},'SLDataType',{'SS_DOUBLE','SS_DOUBLE','SS_DOUBLE','SS_DOUBLE','SS_DOUBLE','SS_DOUBLE','SS_DOUBLE','SS_DOUBLE'}),'StatusSelected','yes','TimeSelected','yes','DeltaTimeSelected','yes','DelayTimeSelected','yes','DelayTimeTXCommandSelected','no','EncodeSetUnusedBitsToOne','no','EnableMsgLoopback','no','TriggerPort',struct('Selected','no','TriggerType',0),'EnablePortSelected','yes','UserCoding',struct('Selected','yes','InterfaceFile','UserEncodingFile','FcnName','Message_CRC_Encoder','InportSelected','no','InportWidth',1,'OutportSelected','no','OutportWidth',1),'TerminationMsg',struct('Selected','no','Byte0','0x00','Byte1','0x00','Byte2','0x00','Byte3','0x00','Byte4','0x00','Byte5','0x00','Byte6','0x00','Byte7','0x00'),'InitialMsg',struct('Selected','no','Byte0','0x00','Byte1','0x00','Byte2','0x00','Byte3','0x00','Byte4','0x00','Byte5','0x00','Byte6','0x00','Byte7','0x00'),'BoardType','DS1','BoardNo',1,'ControllerNo',2),'OFF',[]}},'TLCFileName',{{'rtican_tx_message','OFF',[]}})  RTISFcnParameters=struct('SFcnRTICANMessage','struct','TLCFileName','char')  RTIBlockParaDefault=struct('BoardTypeNo',4302,'BoardNo',1,'ChannelNo',1,'Parameters',struct('DataFileSupport',struct('DataFileSelectedMaster',0,'DataFileSelectedLocal',0,'DataFileName','','DataFileDate','','SelectedFile',['<no file selected>']),'Options',struct('StatusSelected',1,'TimeSelected',1,'DeltaTimeSelected',1,'DelayTimeSelected',1,'DelayTimeTXCommandSelected',0,'EncodeSetUnusedBitsToOne',0,'EnableMsgLoopback',0,'TriggerPort',struct('Selected',0,'TriggerType','rising'),'EnablePortSelected',0,'SignalOnPortnameSelected',1,'UserCoding',struct('Selected',0,'InterfaceFile','UserEncodingFile','FcnName','UserEncodeFcn','InportSelected',0,'InportWidth',1,'OutportSelected',0,'OutportWidth',1),'TerminationMsg',struct('Selected',0,'Byte0_7','0'),'InitialMsg',struct('Selected',0,'Byte0_7','0')),'Message',struct('MsgOnBlocknameSelected',0,'MsgName',['TX Message'],'MsgIdFormat',0,'MsgId',100,'MsgLength',8,'NumSignals',1,'SampleTime',-1,'StartTime',struct('Selected',0,'Value',0),'AutoRepeatTime',struct('Selected',0,'Value',0.1),'Timeout',struct('Selected',0,'Value',0.1),'DelayTime',struct('Selected',0,'Value',0.1),'Signal',struct('SgnName',['TX signal'],'SgnStartBit',0,'SgnLength',8,'SgnType',0,'ModeValue',-1,'DataType',0,'SLDataType','SS_DOUBLE','ByteLayout',0,'Factor',1,'Offset',0,'Min',0,'Max',255,'SgnComment',{{}},'SgnUnit',''),'MsgIdNumFormat',0,'MsgComment',{{''}}),'Version',1.2,'general',struct('isFromLib',1)),'GroupId',struct('Group',{{'RTICAN'}},'No',1,'Behavior',{{'NAMECHANGE'}},'BlockType',{{'SINK'}},'NameChangeFlag',0),'SFcnRTICANMessage',struct('MsgType','TX','MsgName',['TX Message'],'MsgIdFormat','STD','MsgId',100,'MsgLength',2,'NumSignals',1,'SampleTime',-1,'StartTime',struct('Selected','no','Value',0),'AutoRepeatTime',struct('Selected','no','Value',0.1),'Timeout',struct('Selected','no','Value',0.1),'DelayTime',struct('Selected','no','Value',0.1),'Signal',struct('SgnName',['TX signal'],'SgnStartBit',0,'SgnLength',8,'SgnType','standard','ModeValue',-1,'DataType',['unsigned int'],'ByteLayout',['little endian'],'SLDataType','SS_DOUBLE','Factor',1,'Offset',0),'StatusSelected','yes','TimeSelected','yes','DeltaTimeSelected','yes','DelayTimeSelected','yes','EnablePortSelected','no','EnableMsgLoopback','no','DelayTimeTXCommandSelected','no','EncodeSetUnusedBitsToOne','no','UserCoding',struct('Selected','no','InterfaceFile','UserDecodingFile','FcnName','UserDecodeFcn','InportSelected','no','InportWidth',1,'OutportSelected','no','OutportWidth',1),'TerminationMsg',struct('Selected','no','Byte0','0x00','Byte1','0x00','Byte2','0x00','Byte3','0x00','Byte4','0x00','Byte5','0x00','Byte6','0x00','Byte7','0x00'),'InitialMsg',struct('Selected','no','Byte0','0x00','Byte1','0x00','Byte2','0x00','Byte3','0x00','Byte4','0x00','Byte5','0x00','Byte6','0x00','Byte7','0x00'),'TriggerPort',struct('Selected','no','TriggerType','rising'),'BoardType','DS4302','BoardNo',1,'ControllerNo',1,'SFcnPortType','Scalar'),'TLCFileName','rtican_tx_message')
      settings: AttributesFormatString=Group Id: RTICAN2\n  SourceProductName=dSPACE RTI CAN Blockset
  Data Type Conversion1 : DataTypeConversion  OutDataTypeStr=double
  Long_Accel_sds_mot_ref : Constant  Value=2077  OutMin=0  OutMax=5000  OutDataTypeStr=Inherit: Inherit via back propagation
  SDS_Motion_Ref : rtican/RTICAN Transmit (TX)   Reserved1=[]  Reserved2=[]  Reserved3=[]  Reserved4=[]  SfcnMessage=[]  Msg_Struct=[]  BoardTypeNo=[]  BoardNo=[]  ChannelNo=[]  Parameters=[]  DialogFcn=[]  UnitName=[]  Revision=[]  UnitValues=[]  DSProperties=struct('RTI',struct('Version',uint32(5),'BlockType',struct('isSLSource',uint8(1),'isSLSink',uint8(1),'isHWSource',uint8(0),'isHWSink',uint8(0),'isSetup',uint8(0),'isInline',uint8(1),'isNonInline',uint8(0),'isInterrupt',uint8(0),'isChannelwise',uint8(0)),'IOBoardType','RTICAN','UnitType','MESSAGE','Identifier','TX','DialogType','MSVC','BlockSet','RTICAN','SlaveProcessor','CAN'))  RTIBlockInterface=struct('InputPortsWidth',int32([1 1 1 1]),'InputPortsActive',[1 1 1 1],'InputPortsName',{{'VEH_SPEED','MC_SDS_Motion_Ref','LongAcceleration','CRC_SDS_Motion_Ref'}},'InputPortsDataType',{{'SS_DOUBLE','SS_DOUBLE','SS_DOUBLE','SS_DOUBLE'}},'OutputPortsWidth',int32([1 1 1 1]),'OutputPortsActive',[1 1 1 1],'OutputPortsName',{{['TX status'],['TX time'],['TX delta time'],['TX delay time']}},'DialogFcn','rtican_message_interface_gui','BlockDisplay',{{'','center'}},'IconTransparency','on','InitLevel',3,'BlockName',struct('Token',{{'SDS_Motion_Ref'}}),'SampleTime',{{-1}},'TriggerPort',{{'none'}},'EnablePort',{{'yes'}})  RTIBlockParameters=struct('BoardTypeNo',{{1,'OFF',[]}},'BoardNo',{{1,'ON',[1 16]}},'ChannelNo',{{2,'ON',[1 2]}},'Parameters',{{struct('DataFileSupport',struct('DataFileSelectedMaster',1,'DataFileSelectedLocal',1,'DataFileName',['c:\intrepidcs\pacifica dbc\e4a_r4_ccan3_cr11690_mod.dbc|'],'DataFileDate',{{{['26-Feb-2019 09:24:57']}}},'SelectedFile',['..\..\..\..\..\intrepidcs\pacifica dbc\e4a_r4_ccan3_cr11690_mod.dbc']),'Options',struct('StatusSelected',1,'TimeSelected',1,'DeltaTimeSelected',1,'DelayTimeSelected',1,'DelayTimeTXCommandSelected',0,'EncodeSetUnusedBitsToOne',0,'EnableMsgLoopback',0,'TriggerPort',struct('Selected',0,'TriggerType',0),'EnablePortSelected',1,'SignalOnPortnameSelected',1,'UserCoding',struct('Selected',1,'InterfaceFile','UserEncodingFile','FcnName','Message_CRC_Encoder','InportSelected',0,'InportWidth',1,'OutportSelected',0,'OutportWidth',1),'TerminationMsg',struct('Selected',0,'Byte0_7','0'),'InitialMsg',struct('Selected',0,'Byte0_7','0')),'Message',struct('MsgOnBlocknameSelected',1,'MsgName','SDS_Motion_Ref','MsgIdFormat',0,'MsgId',298,'MsgLength',6,'NumSignals',4,'SampleTime',-1,'StartTime',struct('Selected',1,'Value',0),'AutoRepeatTime',struct('Selected',1,'Value',0.01),'Timeout',struct('Selected',0,'Value',0.1),'DelayTime',struct('Selected',0,'Value',0.1),'Signal',struct('SgnName',{'VEH_SPEED','MC_SDS_Motion_Ref','LongAcceleration','CRC_SDS_Motion_Ref'},'SgnStartBit',{16,36,36,40},'SgnLength',{16,4,12,8},'SgnType',{0,0,0,0},'ModeValue',{-1,-1,-1,-1},'DataType',{0,0,0,0},'ByteLayout',{2,0,2,0},'Factor',{2^-7,1,0.02,1},'Offset',{0,0,-40.96,0},'SgnComment',{{['Vehicle speed']},{['Message counter']},{['Raw longitudinal acceleration']},{['CRC-checksum byte 1 to 4 according to SAE J1850']}},'SgnUnit',{'km/h','','m/s�',''},'Min',{0,0,-40.96,0},'Max',{511.984375,15,40.92,0},'SLDataType',{'SS_DOUBLE','SS_DOUBLE','SS_DOUBLE','SS_DOUBLE'}),'MsgIdNumFormat',0,'MsgComment',{{''}}),'Version',1.2,'general',struct('isFromLib',0)),'OFF',[]}},'GroupId',{{struct('Group',{{'RTICAN'}},'No',2,'Behavior',{{'NAMECHANGE'}},'BlockType',{{'SINK'}},'NameChangeFlag',0),'OFF',[]}},'SFcnRTICANMessage',{{struct('MsgType','TX','SFcnPortType','Scalar','MsgName','SDS_Motion_Ref','MsgIdFormat','STD','MsgId',298,'MsgLength',6,'NumSignals',4,'SampleTime',-1,'StartTime',struct('Selected','yes','Value',0),'AutoRepeatTime',struct('Selected','yes','Value',0.01),'Timeout',struct('Selected','no','Value',0.1),'Signal',struct('SgnName',{'VEH_SPEED','MC_SDS_Motion_Ref','LongAcceleration','CRC_SDS_Motion_Ref'},'SgnStartBit',{16,36,36,40},'SgnLength',{16,4,12,8},'SgnType',{'standard','standard','standard','standard'},'ModeValue',{-1,-1,-1,-1},'DataType',{['unsigned int'],['unsigned int'],['unsigned int'],['unsigned int']},'ByteLayout',{['motorola back.'],['little endian'],['motorola back.'],['little endian']},'Factor',{2^-7,1,0.02,1},'Offset',{0,0,-40.96,0},'SLDataType',{'SS_DOUBLE','SS_DOUBLE','SS_DOUBLE','SS_DOUBLE'}),'StatusSelected','yes','TimeSelected','yes','DeltaTimeSelected','yes','DelayTimeSelected','yes','DelayTimeTXCommandSelected','no','EncodeSetUnusedBitsToOne','no','EnableMsgLoopback','no','TriggerPort',struct('Selected','no','TriggerType',0),'EnablePortSelected','yes','UserCoding',struct('Selected','yes','InterfaceFile','UserEncodingFile','FcnName','Message_CRC_Encoder','InportSelected','no','InportWidth',1,'OutportSelected','no','OutportWidth',1),'TerminationMsg',struct('Selected','no','Byte0','0x00','Byte1','0x00','Byte2','0x00','Byte3','0x00','Byte4','0x00','Byte5','0x00','Byte6','0x00','Byte7','0x00'),'InitialMsg',struct('Selected','no','Byte0','0x00','Byte1','0x00','Byte2','0x00','Byte3','0x00','Byte4','0x00','Byte5','0x00','Byte6','0x00','Byte7','0x00'),'BoardType','DS1','BoardNo',1,'ControllerNo',2),'OFF',[]}},'TLCFileName',{{'rtican_tx_message','OFF',[]}})  RTISFcnParameters=struct('SFcnRTICANMessage','struct','TLCFileName','char')  RTIBlockParaDefault=struct('BoardTypeNo',4302,'BoardNo',1,'ChannelNo',1,'Parameters',struct('DataFileSupport',struct('DataFileSelectedMaster',0,'DataFileSelectedLocal',0,'DataFileName','','DataFileDate','','SelectedFile',['<no file selected>']),'Options',struct('StatusSelected',1,'TimeSelected',1,'DeltaTimeSelected',1,'DelayTimeSelected',1,'DelayTimeTXCommandSelected',0,'EncodeSetUnusedBitsToOne',0,'EnableMsgLoopback',0,'TriggerPort',struct('Selected',0,'TriggerType','rising'),'EnablePortSelected',0,'SignalOnPortnameSelected',1,'UserCoding',struct('Selected',0,'InterfaceFile','UserEncodingFile','FcnName','UserEncodeFcn','InportSelected',0,'InportWidth',1,'OutportSelected',0,'OutportWidth',1),'TerminationMsg',struct('Selected',0,'Byte0_7','0'),'InitialMsg',struct('Selected',0,'Byte0_7','0')),'Message',struct('MsgOnBlocknameSelected',0,'MsgName',['TX Message'],'MsgIdFormat',0,'MsgId',100,'MsgLength',8,'NumSignals',1,'SampleTime',-1,'StartTime',struct('Selected',0,'Value',0),'AutoRepeatTime',struct('Selected',0,'Value',0.1),'Timeout',struct('Selected',0,'Value',0.1),'DelayTime',struct('Selected',0,'Value',0.1),'Signal',struct('SgnName',['TX signal'],'SgnStartBit',0,'SgnLength',8,'SgnType',0,'ModeValue',-1,'DataType',0,'SLDataType','SS_DOUBLE','ByteLayout',0,'Factor',1,'Offset',0,'Min',0,'Max',255,'SgnComment',{{}},'SgnUnit',''),'MsgIdNumFormat',0,'MsgComment',{{''}}),'Version',1.2,'general',struct('isFromLib',1)),'GroupId',struct('Group',{{'RTICAN'}},'No',1,'Behavior',{{'NAMECHANGE'}},'BlockType',{{'SINK'}},'NameChangeFlag',0),'SFcnRTICANMessage',struct('MsgType','TX','MsgName',['TX Message'],'MsgIdFormat','STD','MsgId',100,'MsgLength',2,'NumSignals',1,'SampleTime',-1,'StartTime',struct('Selected','no','Value',0),'AutoRepeatTime',struct('Selected','no','Value',0.1),'Timeout',struct('Selected','no','Value',0.1),'DelayTime',struct('Selected','no','Value',0.1),'Signal',struct('SgnName',['TX signal'],'SgnStartBit',0,'SgnLength',8,'SgnType','standard','ModeValue',-1,'DataType',['unsigned int'],'ByteLayout',['little endian'],'SLDataType','SS_DOUBLE','Factor',1,'Offset',0),'StatusSelected','yes','TimeSelected','yes','DeltaTimeSelected','yes','DelayTimeSelected','yes','EnablePortSelected','no','EnableMsgLoopback','no','DelayTimeTXCommandSelected','no','EncodeSetUnusedBitsToOne','no','UserCoding',struct('Selected','no','InterfaceFile','UserDecodingFile','FcnName','UserDecodeFcn','InportSelected','no','InportWidth',1,'OutportSelected','no','OutportWidth',1),'TerminationMsg',struct('Selected','no','Byte0','0x00','Byte1','0x00','Byte2','0x00','Byte3','0x00','Byte4','0x00','Byte5','0x00','Byte6','0x00','Byte7','0x00'),'InitialMsg',struct('Selected','no','Byte0','0x00','Byte1','0x00','Byte2','0x00','Byte3','0x00','Byte4','0x00','Byte5','0x00','Byte6','0x00','Byte7','0x00'),'TriggerPort',struct('Selected','no','TriggerType','rising'),'BoardType','DS4302','BoardNo',1,'ControllerNo',1,'SFcnPortType','Scalar'),'TLCFileName','rtican_tx_message')
      settings: AttributesFormatString=Group Id: RTICAN2\n  SourceProductName=dSPACE RTI CAN Blockset
  Terminator{1..7,14} (8 alike) : Terminator
  Veh_Speed_sds_mot_ref : Constant  Value=0  OutMin=0  OutMax=6  OutDataTypeStr=Inherit: Inherit via back propagation
  Zero-Order Hold : ZeroOrderHold  SampleTime=-1
  wires:
  DAS_A3_A/1 -> Terminator14/1
  In1/1 -> Bus Creator/1
  In2/1 -> Bus Creator/2
  In3/1 -> Bus Creator/3
  In4/1 -> Bus Creator/4
  In5/1 -> Bus Creator/5
  In6/1 -> Bus Creator/6
  In7/1 -> Bus Creator/7
  In8/1 -> Bus Creator/8
  Bus Creator/1 -> Zero-Order Hold/1
  Zero-Order Hold/1 -> Bus Selector/1
  Bus Selector/1 -> DAS_A3_A/1  "<signal1>"
  Bus Selector/2 -> DAS_A3_A/2  "<signal2>"
  Bus Selector/3 -> DAS_A3_A/3  "<signal3>"
  Bus Selector/4 -> DAS_A3_A/4  "<signal4>"
  Bus Selector/5 -> DAS_A3_A/5  "<signal5>"
  Bus Selector/6 -> DAS_A3_A/6  "<signal6>"
  Bus Selector/7 -> DAS_A3_A/7  "<signal7>"
  Bus Selector/8 -> DAS_A3_A/8  "<signal8>"
  DAS_A3_A/2 -> Terminator1/1
  DAS_A3_A/3 -> Terminator2/1
  DAS_A3_A/4 -> Terminator3/1
  SDS_Motion_Ref/4 -> Terminator7/1
  SDS_Motion_Ref/2 -> Terminator4/1
  SDS_Motion_Ref/1 -> Terminator5/1
  SDS_Motion_Ref/3 -> Terminator6/1
  Counter Limited1/1 -> Data Type Conversion1/1
  Data Type Conversion1/1 -> SDS_Motion_Ref/2
  CRC_SDS_Motion_Ref/1 -> SDS_Motion_Ref/4
  Veh_Speed_sds_mot_ref/1 -> SDS_Motion_Ref/1
  Long_Accel_sds_mot_ref/1 -> SDS_Motion_Ref/3
  In9/1 -> DAS_A3_A/Enable
  In10/1 -> SDS_Motion_Ref/Enable
